simulink model "DualInputVariable"  (R2022a)
settings: Solver=VariableStepAuto  StartTime=0.0  StopTime=0.05  MaxStep=1e-4  RelTol=1e-4  EnableMultiTasking=on
libraries: spsSeriesRLCBranchLib x5, spsVoltageMeasurementLib x4, spsDiodeLib x3, spsMosfetLib x2, spsPWMGeneratorDCDCLib x2, spsControlledVoltageSourceLib x1, eeDcDcVoltageController x1, msbUtilities x1, spsDCVoltageSourceLib x1, spspowerguiLib x1
settings Model: Creator=The MathWorks, Inc.  LastModifiedBy=saturn
settings SolverCC: AlgebraicLoopSolver=TrustRegion  SolverResetMethod=Robust
settings OptimizationCC: EfficientFloat2IntCast=on  LifeSpan=inf
settings DebuggingCC: ReadBeforeWriteMsg=DisableAll  WriteAfterWriteMsg=DisableAll  WriteAfterReadMsg=DisableAll  UnconnectedInputMsg=warning  UnconnectedOutputMsg=warning  UnconnectedLineMsg=warning  UniqueDataStoreMsg=error  StrictBusMsg=ErrorOnBusTreatedAsVector  SFUnexpectedBacktrackingDiag=warning  SFNoUnconditionalDefaultTransitionDiag=warning  SFExecutionAtInitializationDiag=none  SFMachineParentedDataDiag=warning  ArithmeticOperatorsInVariantConditions=warning
settings ModelReferenceCC: UpdateModelReferenceTargets=IfOutOfDate
settings SFSimCC: SFSimEcho=off  SimUseLocalCustomCode=off  CustomCodeUndefinedFunction=UseInterfaceOnly
settings RTWCC: RTWUseLocalCustomCode=off
settings CodeAppCC: StateflowObjectComments=on
settings GRTTargetCC: TargetLangStandard=C89/C90 (ANSI)
settings ConfigComp: CovMetricSettings=dw  CovSaveCumulativeToWorkspaceVar=on  CovSaveSingleToWorkspaceVar=on  CovExternalEMLEnable=off
settings SimscapeCC: SimscapeNormalizeSystem=off  SimscapeNominalValues={1, 'bar'; 1, 'cm^3/s'; 1, 'bar*kg/s'; 1, 'kJ/kg'; 1, 'kW'; }

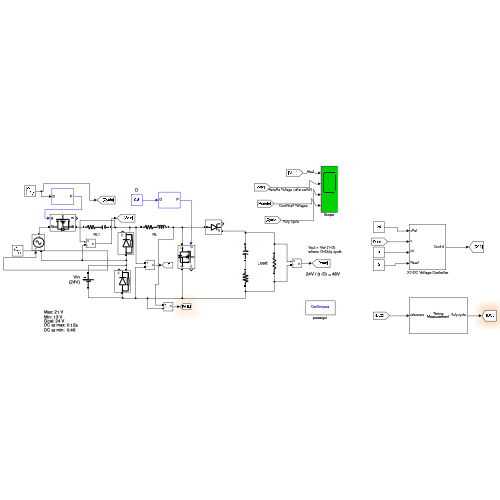
[thumbnail: Simulink's stored preview of the top-level diagram]
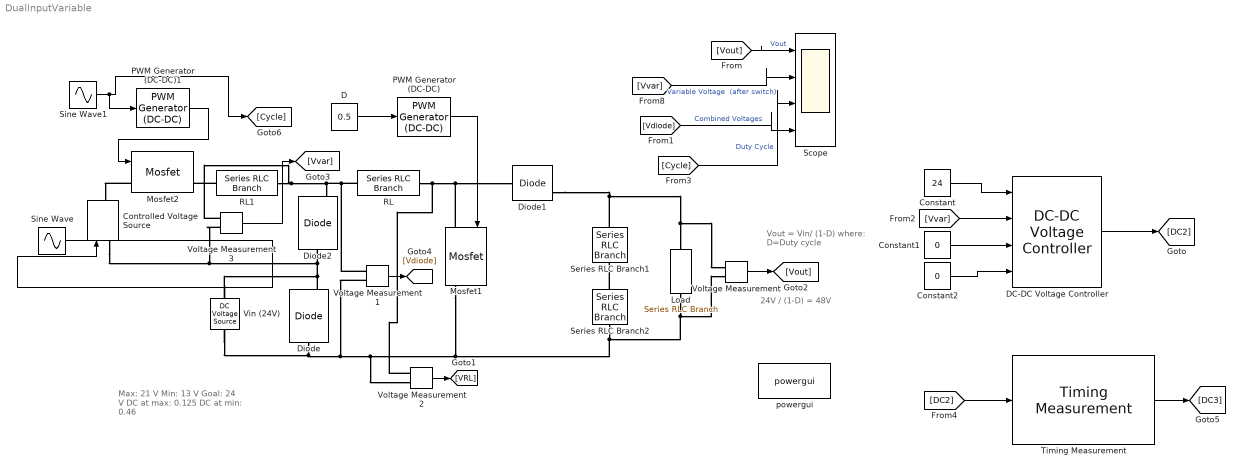
== system DualInputVariable ==
  note: 24V / (1-D) = 48V
  note: Vout = Vin/ (1-D)
      | where: D=Duty cycle
  note: Max: 21 V
      | Min: 13 V
      | Goal: 24 V
      | DC at max: 0.125
      | DC at min: 0.46
  Constant : Constant  Value=24
  Constant1 : Constant  Value=0
  Constant2 : Constant  Value=0
  Controlled Voltage Source : spsControlledVoltageSourceLib/Controlled Voltage Source  Initialize=on  Source_Type=DC  Amplitude=0  Phase=0  Frequency=0  Measurements=Voltage
  D : Constant  Value=0.5
  DC-DC Voltage Controller : eeDcDcVoltageController/DC-DC Voltage Controller  Kp=0.1  Ki=50  Kaw=1  up=1  lo=0  Ts=-1  Tf=0.0001  ActVdcFilter=on
      settings: SourceProductBaseCode=PS
  Diode : spsDiodeLib/Diode  Ron=0.001  Lon=0  Vf=0.8  IC=0  UseSnubber=0  Rs=500  Cs=250e-9  Measurements=on
  Diode1 : spsDiodeLib/Diode  Ron=1e-3  Lon=0  Vf=0  IC=0  UseSnubber=off  Rs=inf  Cs=inf  Measurements=on
  Diode2 : spsDiodeLib/Diode  Ron=0.001  Lon=0  Vf=0.8  IC=0  UseSnubber=0  Rs=500  Cs=250e-9  Measurements=on
  Load : spsSeriesRLCBranchLib/Series RLC Branch  LConnTagsString=__new0  RConnTagsString=__new0  BranchType=R  Resistance=3  Inductance=200e-6  SetiL0=off  InitialCurrent=0  Capacitance=400e-6  Setx0=off  InitialVoltage=0  Measurements=None
  Mosfet1 : spsMosfetLib/Mosfet  Ron=1e-3  Lon=0  Rd=1e-3  Vfd=0  IC=0  Rs=inf  Cs=inf  Measurements=on
  Mosfet2 : spsMosfetLib/Mosfet  Ron=1e-3  Lon=0  Rd=1e-3  Vfd=0  IC=0  Rs=inf  Cs=inf  Measurements=on
  PWM Generator (DC-DC) : spsPWMGeneratorDCDCLib/PWM Generator (DC-DC)  Fsw=20e3  Ts=0
  PWM Generator (DC-DC)1 : spsPWMGeneratorDCDCLib/PWM Generator (DC-DC)  Fsw=150e3  Ts=0
  RL : spsSeriesRLCBranchLib/Series RLC Branch  LConnTagsString=__new0  RConnTagsString=__new0  BranchType=RL  Resistance=1e-3  Inductance=250e-6  SetiL0=off  InitialCurrent=0  Capacitance=1e-6  Setx0=off  InitialVoltage=0  Measurements=None
  RL1 : spsSeriesRLCBranchLib/Series RLC Branch  LConnTagsString=__new0  RConnTagsString=__new0  BranchType=RC  Resistance=1e-3  Inductance=250e-6  SetiL0=off  InitialCurrent=0  Capacitance=1e-6  Setx0=off  InitialVoltage=0  Measurements=None
  Scope : Scope  NumInputPorts=4
  Series RLC Branch1 : spsSeriesRLCBranchLib/Series RLC Branch  LConnTagsString=__new0  RConnTagsString=__new0  BranchType=C  Resistance=1e-4  Inductance=200e-6  SetiL0=off  InitialCurrent=0  Capacitance=200e-6  Setx0=off  InitialVoltage=40  Measurements=None
  Series RLC Branch2 : spsSeriesRLCBranchLib/Series RLC Branch  LConnTagsString=__new0  RConnTagsString=__new0  BranchType=R  Resistance=1e-4  Inductance=200e-6  SetiL0=off  InitialCurrent=0  Capacitance=200e-6  Setx0=off  InitialVoltage=40  Measurements=None
  Sine Wave : Sin  Amplitude=4  Bias=17  Frequency=1000  SampleTime=0
  Sine Wave1 : Sin  Amplitude=0.1  Bias=0.2925  Frequency=1000  Phase=3  SampleTime=0
  Timing Measurement : msbUtilities/Timing Measurement  Period=off  Frequency=off  RiseTime=off  FallTime=off  DutyCycle=on  Delay=off  SameRefThreshold=on  GlobalRefThreshold=0  Range=[-1 1]  MeasurementType=80% / 20%  ThresholdMax=0.6  ThresholdMin=-0.6  DcRefThreshold=0  DelayRefThreshold=0  DelayTstThreshold=0
      settings: SourceProductBaseCode=AM
  Vin (24V) : spsDCVoltageSourceLib/DC Voltage Source  Amplitude=24  Measurements=None
  Voltage Measurement{,1..3} (4 alike) : spsVoltageMeasurementLib/Voltage Measurement  PhasorSimulation=off  OutputType=Complex  PSBequivalent=0
  powergui : spspowerguiLib/powergui  Priority=1  SimulationMode=Continuous  SampleTime=50e-6  frequency=60  Iterations=50  frequencyindice=0  Pbase=100e6  ErrMax=1e-4  UnitsV=kV  UnitsW=MW  buscounter=0  FunctionMessages=off  echomessages=off  EnableUseOfTLC=off  CurrentSourceSwitches=off  DisableSnubberDevices=off  DisableRonSwitches=off  DisableVfSwitches=off  DisplayEquations=off  AutomaticDiscreteSolvers=off  SolverType=Tustin/Backward Euler (TBE)  Interpol=off  ExternalGateDelay=off  methode=off  Ts=100  x0status=blocks  SPID=on  SwTol=0  HookPort=off  NonlinearTolerance=1e-4  nMaxIteration=100  ContinueOnMaxIteration=off  RestoreLinks=warning  ResistiveCurrentMeasurement=off  Frange=[0:2:500]  Ylog=off  Xlog=on  ShowGrid=off  save=off  variable=ZData  structure=0  ZoomFFT=off  StartTime=0.0  cycles=1  DisplayStyle=1  fundamental=60  FreqAxis=off  MaxFrequency=1000  frequencyindicesteady=1  RmsSteady=1  display=off
  wires:
  Voltage Measurement/1 -> [Vout]
  [Vvar] -> Scope/2  "Variable Voltage  (after switch)"
  [Vout] -> Scope/1  "Vout"
  D/1 -> PWM Generator (DC-DC)/1
  Voltage Measurement1/1 -> [Vdiode]
  Voltage Measurement2/1 -> [VRL]
  [Vdiode] -> Scope/4  "Combined Voltages"
  Sine Wave/1 -> Controlled Voltage Source/1
  Voltage Measurement3/1 -> [Vvar]
  [Vvar] -> DC-DC Voltage Controller/2
  Constant/1 -> DC-DC Voltage Controller/1
  Constant1/1 -> DC-DC Voltage Controller/3
  Constant2/1 -> DC-DC Voltage Controller/4
  DC-DC Voltage Controller/1 -> [DC2]
  PWM Generator (DC-DC)/1 -> Mosfet1/1
  [DC2] -> Timing Measurement/1
  Timing Measurement/1 -> [DC3]
  Sine Wave1/1 -> PWM Generator (DC-DC)1/1, [Cycle]
  PWM Generator (DC-DC)1/1 -> Mosfet2/1
  [Cycle] -> Scope/3  "Duty Cycle"
  connections:
  Load/RConn1 -- Series RLC Branch2/RConn1 -- Voltage Measurement2/LConn2 -- Voltage Measurement1/LConn2 -- Vin (24V)/LConn1 -- Diode/LConn1 -- Mosfet1/RConn1 -- Voltage Measurement/LConn2
  Series RLC Branch1/LConn1 -- Diode1/RConn1 -- Voltage Measurement/LConn1 -- Load/LConn1
  RL/RConn1 -- Voltage Measurement2/LConn1 -- Mosfet1/LConn1 -- Diode1/LConn1
  Vin (24V)/RConn1 -- Diode/RConn1 -- Controlled Voltage Source/LConn1 -- Voltage Measurement3/LConn2 -- Diode2/LConn1
  Diode2/RConn1 -- Voltage Measurement3/LConn1 -- RL1/RConn1 -- RL/LConn1 -- Voltage Measurement1/LConn1
  Series RLC Branch2/LConn1 -- Series RLC Branch1/RConn1
  Mosfet2/LConn1 -- Controlled Voltage Source/RConn1
  RL1/LConn1 -- Mosfet2/RConn1
